simulink library "csu_lns_ln200_software_lib_a"  (R2014b)
settings: Solver=ode45  SolverMode=SingleTasking  StartTime=0.0  StopTime=10.0  RelTol=1e-3
values from neighbouring files (symbols this model uses):
  lns_accel_to_count = 1.0/(lns_accel_lsb)    (= 16384)    [csu_lns_ln200_software_init_a.m]
  lns_gyro_to_count = 1.0/(lns_gyro_lsb)    (= 524288)    [csu_lns_ln200_software_init_a.m]
  lns_sample_time = .0025    (= 0.0025)    [csu_lns_ln200_software_init_a.m]
settings Model: Creator=hcannon  LastModifiedBy=mstewart

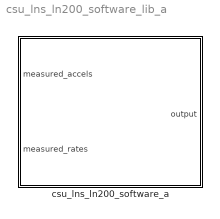
== system csu_lns_ln200_software_lib_a ==
  csu_lns_ln200_software_a : Subsystem  TreatAsAtomicUnit=on

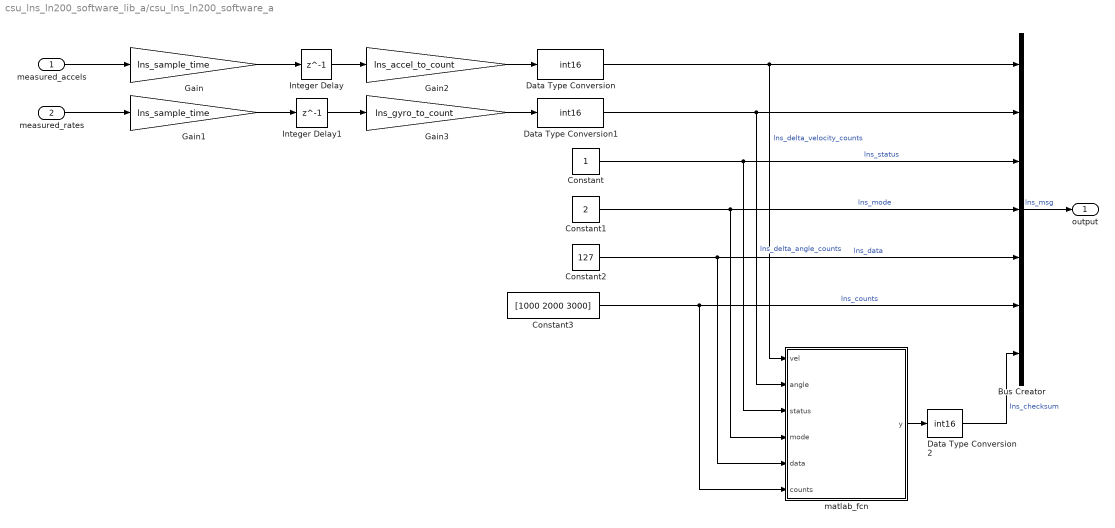
== system csu_lns_ln200_software_lib_a/csu_lns_ln200_software_a ==
  measured_accels : Inport
  measured_rates : Inport  Port=2
  Bus Creator : BusCreator  Inputs=7
  Constant : Constant  OutDataTypeStr=int16
  Constant1 : Constant  Value=2  OutDataTypeStr=int16
  Constant2 : Constant  Value=127  OutDataTypeStr=int16
  Constant3 : Constant  Value=[1000 2000 3000]  OutDataTypeStr=int16
  Data Type Conversion : DataTypeConversion  OutDataTypeStr=int16  RndMeth=Nearest
  Data Type Conversion1 : DataTypeConversion  OutDataTypeStr=int16  RndMeth=Nearest
  Data Type Conversion2 : DataTypeConversion  OutDataTypeStr=int16  RndMeth=Nearest
  Gain : Gain  Gain=lns_sample_time
  Gain1 : Gain  Gain=lns_sample_time
  Gain2 : Gain  Gain=lns_accel_to_count
  Gain3 : Gain  Gain=lns_gyro_to_count
  Integer Delay : Delay  DelayLength=1  InputProcessing=Inherited
  Integer Delay1 : Delay  DelayLength=1  InputProcessing=Inherited
  matlab_fcn : MATLAB Function  TreatAsAtomicUnit=on
  output : Outport
  wires:
  measured_accels/1 -> Gain/1
  measured_rates/1 -> Gain1/1
  Gain/1 -> Integer Delay/1
  Integer Delay/1 -> Gain2/1
  Gain1/1 -> Integer Delay1/1
  Integer Delay1/1 -> Gain3/1
  Gain2/1 -> Data Type Conversion/1
  Gain3/1 -> Data Type Conversion1/1
  matlab_fcn/1(y) -> Data Type Conversion2/1
  Data Type Conversion/1 -> Bus Creator/1, matlab_fcn/1(vel)  "lns_delta_velocity_counts"
  Data Type Conversion1/1 -> Bus Creator/2, matlab_fcn/2(angle)  "lns_delta_angle_counts"
  Constant/1 -> Bus Creator/3, matlab_fcn/3(status)  "lns_status"
  Constant1/1 -> Bus Creator/4, matlab_fcn/4(mode)  "lns_mode"
  Constant2/1 -> Bus Creator/5, matlab_fcn/5(data)  "lns_data"
  Constant3/1 -> Bus Creator/6, matlab_fcn/6(counts)  "lns_counts"
  Bus Creator/1 -> output/1  "lns_msg"
  Data Type Conversion2/1 -> Bus Creator/7  "lns_checksum"

== matlab function csu_lns_ln200_software_lib_a/csu_lns_ln200_software_a/matlab_fcn ==
  data: vel input; y output; angle input; status input; mode input; data input; counts input
function y = calc_checksum(vel,angle,status,mode,data,counts)
% This block supports the Embedded MATLAB subset.
% See the help menu for details. 


y=-(sum(vel)+sum(angle)+sum(status)+sum(mode)+sum(data)+sum(counts)+1);



%temp=sum(vel)+sum(angle)+sum(status)+sum(mode)+sum(data)+sum(counts);
%if(temp<0)
%    temp=temp+65536;
%end
%lsb=mod(temp,256);
%msb=floor(temp/256);
%y=lsb+msb;
%y=mod(y,256);
